simulink model "INS"  (R2018b)
settings: configuration reference "ins_config" (kept outside this file)
undefined symbols (not defined in the file): DiscIntNeverNeededParam, INS_CONST, INS_EXPORT, INS_PARAM
libraries: simulink x99, AP_Math x15, Filter x6, Quaternion x2, Rotation x2
(part 3 of 4)

== system INS/Data_Fusion/AHRS/Correct/Bias_Correction/Onground_Correction ==
  gyr_B_radPs : Inport
  standstill : Inport  Port=2
  Gain : Gain  Gain=2  OutDataTypeStr=single
  Logical Operator : Logic  Operator=NOT  AllPortsSameDT=off  OutDataTypeStr=boolean
  Product : Product  Inputs=3
  Rate Limiter : RateLimiter  RisingSlewLimit=1/600  FallingSlewLimit=-1/3  SampleTimeMode=inherited  InitialCondition=2
  Saturation : Saturate  UpperLimit=1  LowerLimit=1/20
  Saturation1 : Saturate  UpperLimit=3/180*pi  LowerLimit=-3/180*pi
  gyr_bias : Outport
  wires:
  Saturation1/1 -> Product/1
  Gain/1 -> Rate Limiter/1
  Saturation/1 -> Product/3
  Logical Operator/1 -> Gain/1
  gyr_B_radPs/1 -> Saturation1/1
  Product/1 -> gyr_bias/1
  Rate Limiter/1 -> Saturation/1
  standstill/1 -> Product/2, Logical Operator/1

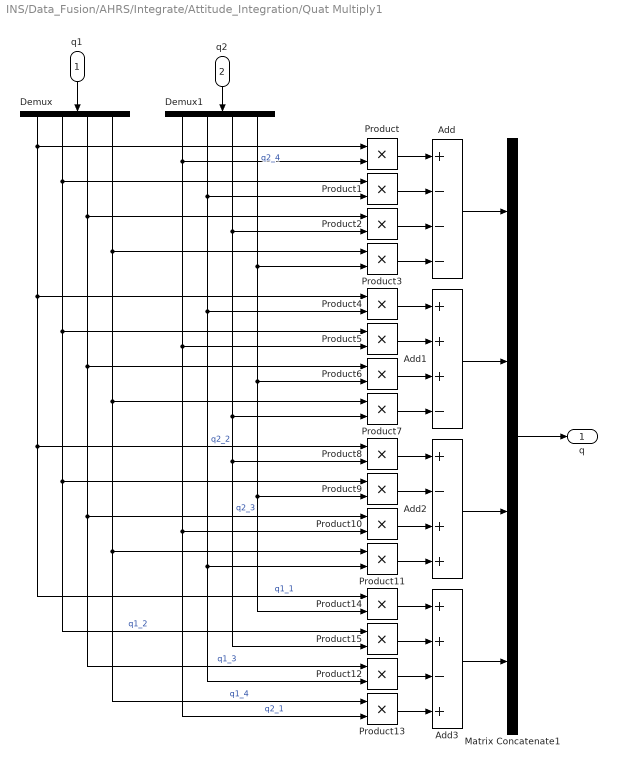
== system INS/Data_Fusion/AHRS/Integrate/Attitude_Integration/Quat Multiply1 ==
  q1 : Inport
  q2 : Inport  Port=2
  Add : Sum  Inputs=+---
  Add1 : Sum  Inputs=+++-
  Add2 : Sum  Inputs=+-++
  Add3 : Sum  Inputs=++-+
  Demux : Demux
  Demux1 : Demux
  Matrix Concatenate1 : Concatenate  NumInputs=4  Mode=Multidimensional array
  Product{,1..15} (16 alike) : Product  RndMeth=Zero
  q : Outport
  wires:
  q1/1 -> Demux/1
  q2/1 -> Demux1/1
  Matrix Concatenate1/1 -> q/1
  Add/1 -> Matrix Concatenate1/1
  Product/1 -> Add/1
  Product1/1 -> Add/2
  Product2/1 -> Add/3
  Product3/1 -> Add/4
  Add1/1 -> Matrix Concatenate1/2
  Product4/1 -> Add1/1
  Product5/1 -> Add1/2
  Product6/1 -> Add1/3
  Product7/1 -> Add1/4
  Product8/1 -> Add2/1
  Product9/1 -> Add2/2
  Product10/1 -> Add2/3
  Product11/1 -> Add2/4
  Product14/1 -> Add3/1
  Product15/1 -> Add3/2
  Product12/1 -> Add3/3
  Product13/1 -> Add3/4
  Add3/1 -> Matrix Concatenate1/4
  Add2/1 -> Matrix Concatenate1/3
  Demux/1 -> Product/1, Product14/1, Product8/1, Product4/1  "q1_1"
  Demux/2 -> Product15/1, Product9/1, Product5/1, Product1/1  "q1_2"
  Demux/3 -> Product12/1, Product10/1, Product6/1, Product2/1  "q1_3"
  Demux/4 -> Product13/1, Product11/1, Product7/1, Product3/1  "q1_4"
  Demux1/4 -> Product14/2, Product9/2, Product6/2, Product3/2  "q2_4"
  Demux1/3 -> Product15/2, Product8/2, Product7/2, Product2/2  "q2_3"
  Demux1/2 -> Product12/2, Product11/2, Product4/2, Product1/2  "q2_2"
  Demux1/1 -> Product13/2, Product10/2, Product5/2, Product/2  "q2_1"

== system INS/Data_Fusion/AHRS/Integrate/Euler_Angle/Euler_Transformations ==
  Oz_B : Inport
  quat_OB : Inport  Port=2
  Demux2 : Demux  Outputs=3
  Gain5 : Gain  Gain=-1
  Saturation1 : Saturate  UpperLimit=0.999  LowerLimit=-0.999
  Trigonometric Function : Trigonometry  Operator=asin
  Trigonometric Function1 : Trigonometry  Operator=atan2
  quat_to_psi : Subsystem
  phi_rad : Outport
  theta_rad : Outport  Port=2
  psi_rad : Outport  Port=3
  wires:
  quat_OB/1 -> quat_to_psi/1(quat)
  Saturation1/1 -> Trigonometric Function/1
  Demux2/1 -> Gain5/1
  Demux2/3 -> Trigonometric Function1/2
  Gain5/1 -> Saturation1/1
  Oz_B/1 -> Demux2/1
  Demux2/2 -> Trigonometric Function1/1
  Trigonometric Function/1 -> theta_rad/1  "theta_rad"
  Trigonometric Function1/1 -> phi_rad/1  "phi_rad"
  quat_to_psi/1(psi) -> psi_rad/1

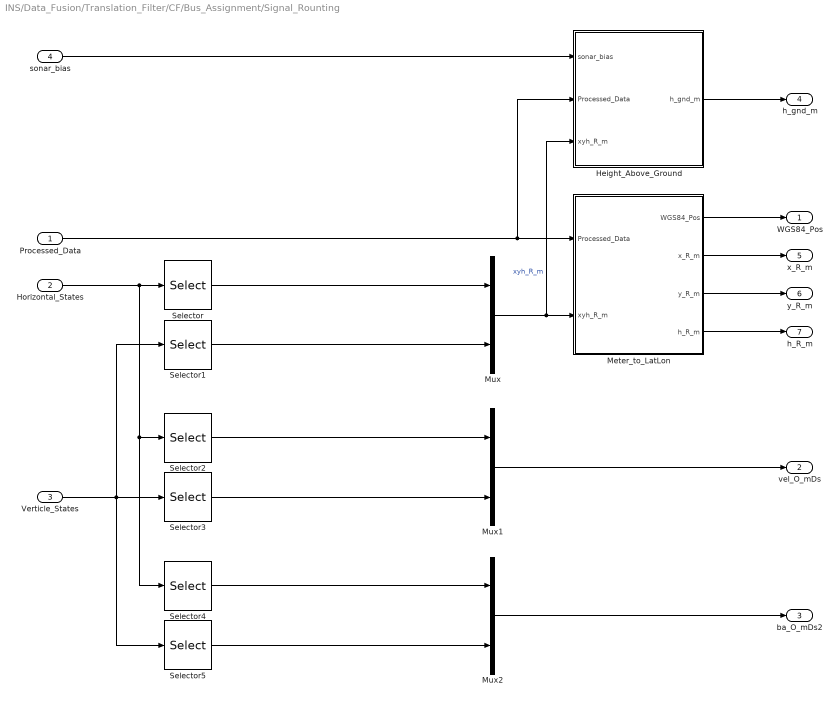
== system INS/Data_Fusion/Translation_Filter/CF/Bus_Assignment/Signal_Rounting ==
  Processed_Data : Inport
  Horizontal_States : Inport  Port=2
  Verticle_States : Inport  Port=3
  sonar_bias : Inport  Port=4
  Height_Above_Ground : Subsystem
  Meter_to_LatLon : Subsystem
  Mux : Mux  Inputs=2
  Mux1 : Mux  Inputs=2
  Mux2 : Mux  Inputs=2
  Selector : Selector  InputPortWidth=6  IndexOptions=Index vector (dialog)  Indices=[1 2]  OutputSizes=1
  Selector1 : Selector  InputPortWidth=3  IndexOptions=Index vector (dialog)  Indices=[1]  OutputSizes=1
  Selector2 : Selector  InputPortWidth=6  IndexOptions=Index vector (dialog)  Indices=[3 4]  OutputSizes=1
  Selector3 : Selector  InputPortWidth=3  IndexOptions=Index vector (dialog)  Indices=[2]  OutputSizes=1
  Selector4 : Selector  InputPortWidth=6  IndexOptions=Index vector (dialog)  Indices=[5 6]  OutputSizes=1
  Selector5 : Selector  InputPortWidth=3  IndexOptions=Index vector (dialog)  Indices=[3]  OutputSizes=1
  WGS84_Pos : Outport
  vel_O_mDs : Outport  Port=2
  ba_O_mDs2 : Outport  Port=3
  h_gnd_m : Outport  Port=4
  x_R_m : Outport  Port=5
  y_R_m : Outport  Port=6
  h_R_m : Outport  Port=7
  wires:
  Mux/1 -> Height_Above_Ground/3(xyh_R_m), Meter_to_LatLon/2(xyh_R_m)  "xyh_R_m"
  Meter_to_LatLon/1(WGS84_Pos) -> WGS84_Pos/1
  Processed_Data/1 -> Height_Above_Ground/2(Processed_Data), Meter_to_LatLon/1(Processed_Data)
  Selector/1 -> Mux/1
  Mux2/1 -> ba_O_mDs2/1
  Selector1/1 -> Mux/2
  Selector4/1 -> Mux2/1
  Selector2/1 -> Mux1/1
  Selector3/1 -> Mux1/2
  Mux1/1 -> vel_O_mDs/1
  Horizontal_States/1 -> Selector/1, Selector2/1, Selector4/1
  Selector5/1 -> Mux2/2
  Verticle_States/1 -> Selector3/1, Selector5/1, Selector1/1
  Height_Above_Ground/1(h_gnd_m) -> h_gnd_m/1
  sonar_bias/1 -> Height_Above_Ground/1(sonar_bias)
  Meter_to_LatLon/4(h_R_m) -> h_R_m/1
  Meter_to_LatLon/2(x_R_m) -> x_R_m/1
  Meter_to_LatLon/3(y_R_m) -> y_R_m/1

== system INS/Data_Fusion/Translation_Filter/CF/Horizontal_Filter/Correct ==
  X_Predict : Inport
  Processed_Data : Inport  Port=2
  Bus Selector : BusSelector  OutputSignals=Sensor_Enable.gps_enable
  GPS_Correct : Subsystem
  Switch : Switch  Criteria=u2 > Threshold
  X_Next : Outport
  wires:
  X_Predict/1 -> GPS_Correct/2(X_Predict), Switch/3
  Processed_Data/1 -> GPS_Correct/1(Processed_Data), Bus Selector/1
  Bus Selector/1 -> GPS_Correct/Enable, Switch/2  "<gps_enable>"
  Switch/1 -> X_Next/1
  GPS_Correct/1(X_Next) -> Switch/1

== system INS/Data_Fusion/Translation_Filter/CF/Horizontal_Filter/Predict ==
  X_Prio : Inport
  Rotation_Data : Inport  Port=2
  Processed_Data : Inport  Port=3
  Propagate : Subsystem
  Update : Subsystem
  X_Predict : Outport
  wires:
  X_Prio/1 -> Propagate/1(X_prio)
  Processed_Data/1 -> Propagate/2(Processed_Data)
  Propagate/1(X) -> Update/1(X_Prio)
  Rotation_Data/1 -> Update/2(Rotation_Data)
  Update/1(X_Predict) -> X_Predict/1

== system INS/Data_Fusion/Translation_Filter/CF/Verticle_Filter/Correct ==
  X_Predict : Inport
  Processed_Data : Inport  Port=2
  Baro_Correct : Subsystem
  GPS_Correct : Subsystem
  X_Next : Outport
  wires:
  Processed_Data/1 -> GPS_Correct/2(Processed_Data), Baro_Correct/2(Processed_Data)
  X_Predict/1 -> Baro_Correct/1(X_Predict)
  Baro_Correct/1(X_Next) -> GPS_Correct/1(X_Predict)
  GPS_Correct/1(X_Next) -> X_Next/1

== system INS/Data_Fusion/Translation_Filter/CF/Verticle_Filter/Predict ==
  X_Prio : Inport
  Rotation_Data : Inport  Port=2
  Processed_Data : Inport  Port=3
  Propagate : Subsystem
  Update : Subsystem
  X_Predict : Outport
  wires:
  X_Prio/1 -> Propagate/1(X_Prio)
  Processed_Data/1 -> Propagate/2(Processed_Data)
  Propagate/1(X) -> Update/1(X_Prio)
  Rotation_Data/1 -> Update/2(Rotation_Data)
  Update/1(X_Predict) -> X_Predict/1

== system INS/Data_Fusion/Translation_Filter/Process/Process_Data/Init_Condition ==
  Validity : Inport
  global_reset : Inport  Port=2
  Sensor_Meas : Inport  Port=3
  Rotation_Data : Inport  Port=4
  Translation_Data : Inport  Port=5
  Bus Creator : BusCreator  Inputs=4
  Bus_Selection : Subsystem
  Pos_Reset : Subsystem
  WGS84_Reference : Subsystem
  Init_Condition : Outport
  wires:
  WGS84_Reference/1(WGS84_Ref) -> Bus Creator/3  "WGS84_Ref"
  Rotation_Data/1 -> Pos_Reset/1(Rotation_Data)
  Bus_Selection/2(WGS84_position) -> WGS84_Reference/4(WGS84_position)
  Bus_Selection/1(WGS84_derivatives) -> WGS84_Reference/3(WGS84_derivatives)
  Pos_Reset/1(pos_reset) -> Bus Creator/1  "pos_reset"
  Sensor_Meas/1 -> Bus_Selection/1(Sensor_Meas)
  Validity/1 -> Pos_Reset/3(Validity), Bus Creator/4, WGS84_Reference/1(Validity)  "Pos_Validity"
  global_reset/1 -> Pos_Reset/2(global_reset)
  Pos_Reset/2(height_reset) -> Bus Creator/2  "height_reset"
  Bus Creator/1 -> Init_Condition/1
  Translation_Data/1 -> WGS84_Reference/2(Translation_Data)

== system INS/Data_Fusion/Translation_Filter/Process/Process_Data/Sensor_Enable ==
  Sensor_Status : Inport
  Bus Creator : BusCreator  Inputs=5
  Bus Selector : BusSelector  OutputSignals=GPS_Status.pos_quality,GPS_Status.spd_quality,GPS_Status.GPS_vaid,OptFlow_Status.opt_flow_valid,Sonar_Status.sonar_valid,Baro_Status.baro_valid
  Sensor_Horizontal_Select : Subsystem
  Sensor_Vertical_Select : Subsystem
  Sensor_Enable : Outport
  wires:
  Bus Selector/3 -> Sensor_Vertical_Select/3(gps_valid), Sensor_Horizontal_Select/3(gps_valid)  "<GPS_vaid>"
  Bus Selector/1 -> Sensor_Vertical_Select/1(gps_pos_quality), Sensor_Horizontal_Select/1(gps_pos_quality)  "<pos_quality>"
  Sensor_Status/1 -> Bus Selector/1
  Sensor_Horizontal_Select/1(gps_enable) -> Bus Creator/1  "gps_enable"
  Sensor_Vertical_Select/2(sonar_enable) -> Bus Creator/4  "sonar_enable"
  Sensor_Vertical_Select/1(gps_hgt_enable) -> Bus Creator/3  "gps_height_enable"
  Bus Creator/1 -> Sensor_Enable/1
  Sensor_Vertical_Select/3(baro_enable) -> Bus Creator/5  "baro_enable"
  Bus Selector/4 -> Sensor_Horizontal_Select/4(opt_flow_valid)  "<opt_flow_valid>"
  Sensor_Horizontal_Select/2(op_flow_enable) -> Bus Creator/2  "opt_flow_enable"
  Bus Selector/2 -> Sensor_Vertical_Select/2(gps_spd_quality), Sensor_Horizontal_Select/2(gps_spd_quality)  "<spd_quality>"
  Bus Selector/6 -> Sensor_Vertical_Select/5(baro_valid)  "<baro_valid>"
  Bus Selector/5 -> Sensor_Vertical_Select/4(sonar_valid)  "<sonar_valid>"

== system INS/Data_Fusion/Translation_Filter/Process/Process_Data/Sensor_Valid ==
  Sensor_Status : Inport
  Bus Creator : BusCreator  Inputs=4
  Position_Validity : Subsystem
  Validity : Outport
  wires:
  Sensor_Status/1 -> Position_Validity/1(Sensor_Status)
  Position_Validity/1(lon_lat_valid) -> Bus Creator/1  "lon_lat_valid"
  Position_Validity/2(xy_R_valid) -> Bus Creator/2  "xy_R_valid"
  Position_Validity/3(altitude_valid) -> Bus Creator/3  "altitude_valid"
  Position_Validity/4(h_R_valid) -> Bus Creator/4  "h_R_valid"
  Bus Creator/1 -> Validity/1

== system INS/Data_Fusion/Translation_Filter/Process/Sensor_Meas/Baro_Process ==
  Sensor_Data : Inport
  Bus Creator : BusCreator  Inputs=2
  Bus Selector1 : BusSelector  OutputSignals=Baro_Data.timestamp,Baro_Data.h_R_m
  Signal Copy : SignalConversion  OverrideOpt=off
  Signal Copy1 : SignalConversion  OverrideOpt=off
  Baro_Meas : Outport
  wires:
  Sensor_Data/1 -> Bus Selector1/1
  Bus Selector1/2 -> Signal Copy1/1  "<h_R_m>"
  Bus Creator/1 -> Baro_Meas/1
  Bus Selector1/1 -> Signal Copy/1  "<timestamp>"
  Signal Copy/1 -> Bus Creator/1  "timestamp_ms"
  Signal Copy1/1 -> Bus Creator/2  "h_R_m"

== system INS/Data_Fusion/Translation_Filter/Process/Sensor_Meas/GPS_Process ==
  Sensor_Data : Inport
  Bus Creator : BusCreator  Inputs=12
  Bus Selector : BusSelector  OutputSignals=GPS_Data.signal6,GPS_Data.signal7,GPS_Data.dz_dh,GPS_Data.mue_rad,GPS_Data.lambda_rad,GPS_Data.height_m,GPS_Data.vn_mPs,GPS_Data.ve_mPs,GPS_Data.vd_mPs,GPS_Data.timestamp_ms,GPS_Data.GPS_reset,GPS_Data.sqd_quality,GPS_Data.pos_quality
  Logical Operator : Logic  Operator=NOT  AllPortsSameDT=off  OutDataTypeStr=boolean
  Multiply : Product
  Multiply1 : Product
  Signal Conversion{,1..9} (10 alike) : SignalConversion  OverrideOpt=off
  GPS_Meas : Outport
  wires:
  Multiply1/1 -> Bus Creator/12  "pos_quality"
  Logical Operator/1 -> Multiply1/1, Multiply/1
  Multiply/1 -> Bus Creator/11  "spd_quality"
  Bus Selector/13 -> Multiply1/2  "<pos_quality>"
  Bus Selector/12 -> Multiply/2  "<sqd_quality>"
  Bus Selector/11 -> Logical Operator/1  "<GPS_reset>"
  Signal Conversion9/1 -> Bus Creator/10  "timestamp_ms"
  Signal Conversion8/1 -> Bus Creator/9  "vel_D_mPs"
  Signal Conversion7/1 -> Bus Creator/8  "vel_E_mPs"
  Signal Conversion6/1 -> Bus Creator/7  "vel_N_mPs"
  Signal Conversion5/1 -> Bus Creator/6  "h_m"
  Signal Conversion4/1 -> Bus Creator/5  "lambda_rad"
  Signal Conversion3/1 -> Bus Creator/4  "mue_rad"
  Signal Conversion2/1 -> Bus Creator/3  "dz_dh"
  Signal Conversion1/1 -> Bus Creator/2  "dy_dlambda"
  Signal Conversion/1 -> Bus Creator/1  "dx_dmue"
  Bus Selector/10 -> Signal Conversion9/1  "<timestamp_ms>"
  Bus Selector/9 -> Signal Conversion8/1  "<vd_mPs>"
  Bus Selector/8 -> Signal Conversion7/1  "<ve_mPs>"
  Bus Selector/7 -> Signal Conversion6/1  "<vn_mPs>"
  Bus Selector/6 -> Signal Conversion5/1  "<height_m>"
  Bus Selector/5 -> Signal Conversion4/1  "<lambda_rad>"
  Bus Selector/4 -> Signal Conversion3/1  "<mue_rad>"
  Bus Selector/3 -> Signal Conversion2/1  "<dz_dh>"
  Bus Selector/2 -> Signal Conversion1/1  "<signal7>"
  Bus Selector/1 -> Signal Conversion/1  "<signal6>"
  Bus Creator/1 -> GPS_Meas/1
  Sensor_Data/1 -> Bus Selector/1

== system INS/Data_Fusion/Translation_Filter/Process/Sensor_Meas/OpticalFlow_Process ==
  Sensor_Data : Inport
  Bus Creator : BusCreator  Inputs=3
  Bus Selector1 : BusSelector  OutputSignals=VisionFlow_Data.timestamp_ms,VisionFlow_Data.vel_x_O_mDs,VisionFlow_Data.vel_y_O_mDs
  Signal Copy : SignalConversion  OverrideOpt=off
  Signal Copy1 : SignalConversion  OverrideOpt=off
  Signal Copy2 : SignalConversion  OverrideOpt=off
  OptFlow_Meas : Outport
  wires:
  Sensor_Data/1 -> Bus Selector1/1
  Bus Creator/1 -> OptFlow_Meas/1
  Signal Copy/1 -> Bus Creator/1  "timestamp_ms"
  Signal Copy1/1 -> Bus Creator/2  "vel_x_O"
  Bus Selector1/1 -> Signal Copy/1  "<timestamp_ms>"
  Bus Selector1/2 -> Signal Copy1/1  "<vel_x_O_mDs>"
  Bus Selector1/3 -> Signal Copy2/1  "<vel_y_O_mDs>"
  Signal Copy2/1 -> Bus Creator/3  "vel_y_O"

== system INS/Data_Fusion/Translation_Filter/Process/Sensor_Meas/Sonar_Process ==
  Sensor_Data : Inport
  Rotation_Data : Inport  Port=2
  Bus Creator : BusCreator  Inputs=2
  Bus Selector : BusSelector  OutputSignals=phi_rad,theta_rad
  Bus Selector1 : BusSelector  OutputSignals=Sonar_Data.timestamp_ms,Sonar_Data.distance_m
  Cos : Trigonometry  Operator=cos
  Cos1 : Trigonometry  Operator=cos
  Multiply : Product  Inputs=3
  Signal Copy : SignalConversion  OverrideOpt=off
  Sonar_Meas : Outport
  wires:
  Rotation_Data/1 -> Bus Selector/1
  Sensor_Data/1 -> Bus Selector1/1
  Bus Selector1/2 -> Multiply/1  "<distance_m>"
  Bus Selector/1 -> Cos/1  "<phi_rad>"
  Bus Selector/2 -> Cos1/1  "<theta_rad>"
  Cos/1 -> Multiply/2
  Cos1/1 -> Multiply/3
  Multiply/1 -> Bus Creator/2  "distance_m"
  Bus Creator/1 -> Sonar_Meas/1
  Bus Selector1/1 -> Signal Copy/1  "<timestamp_ms>"
  Signal Copy/1 -> Bus Creator/1  "timestamp_ms"

== system INS/Data_Fusion/Translation_Filter/Process/Sensor_Status/Baro_Status ==
  Sensor_Data : Inport
  Bus Creator : BusCreator  Inputs=1
  Bus Selector : BusSelector  OutputSignals=Baro_Data.baro_valid
  Signal Conversion1 : SignalConversion  OverrideOpt=off
  Baro_Status : Outport
  wires:
  Bus Selector/1 -> Signal Conversion1/1  "<baro_valid>"
  Bus Creator/1 -> Baro_Status/1
  Sensor_Data/1 -> Bus Selector/1
  Signal Conversion1/1 -> Bus Creator/1  "baro_valid"

== system INS/Data_Fusion/Translation_Filter/Process/Sensor_Status/GPS_Status ==
  Sensor_Data : Inport
  Bus Creator : BusCreator  Inputs=3
  Bus Selector : BusSelector  OutputSignals=GPS_Data.GPS_reset,GPS_Data.sqd_quality,GPS_Data.pos_quality
  Logical Operator : Logic  Operator=NOT  AllPortsSameDT=off  OutDataTypeStr=boolean
  Signal Conversion : SignalConversion  OverrideOpt=off
  Signal Conversion1 : SignalConversion  OverrideOpt=off
  GPS_Status : Outport
  wires:
  Bus Creator/1 -> GPS_Status/1
  Signal Conversion1/1 -> Bus Creator/3  "pos_quality"
  Signal Conversion/1 -> Bus Creator/2  "spd_quality"
  Logical Operator/1 -> Bus Creator/1  "GPS_vaid"
  Bus Selector/3 -> Signal Conversion1/1  "<pos_quality>"
  Bus Selector/2 -> Signal Conversion/1  "<sqd_quality>"
  Bus Selector/1 -> Logical Operator/1  "<GPS_reset>"
  Sensor_Data/1 -> Bus Selector/1

== system INS/Data_Fusion/Translation_Filter/Process/Sensor_Status/OpticalFlow_Status ==
  Sensor_Data : Inport
  Bus Creator : BusCreator  Inputs=1
  Bus Selector : BusSelector  OutputSignals=VisionFlow_Data.valid
  Signal Conversion1 : SignalConversion  OverrideOpt=off
  OptFlow_Status : Outport
  wires:
  Bus Selector/1 -> Signal Conversion1/1  "<valid>"
  Bus Creator/1 -> OptFlow_Status/1
  Sensor_Data/1 -> Bus Selector/1
  Signal Conversion1/1 -> Bus Creator/1  "opt_flow_valid"

== system INS/Data_Fusion/Translation_Filter/Process/Sensor_Status/Sonar_Status ==
  Sensor_Data : Inport
  Bus Creator : BusCreator  Inputs=1
  Bus Selector : BusSelector  OutputSignals=Sonar_Data.sonar_valid
  Signal Conversion1 : SignalConversion  OverrideOpt=off
  Sonar_Status : Outport
  wires:
  Signal Conversion1/1 -> Bus Creator/1  "sonar_valid"
  Sensor_Data/1 -> Bus Selector/1
  Bus Creator/1 -> Sonar_Status/1
  Bus Selector/1 -> Signal Conversion1/1  "<sonar_valid>"

== system INS/Sensor_Process/GPS_Process/GPS_Status_and_Quality/GPS_Status/Init_Condition ==
  valid : Inport
  Compare To Constant3 : simulink/Logic and Bit Operations/Compare To Constant  relop=>=  const=1000  OutDataTypeStr=boolean
  Saturation : Saturate  UpperLimit=2000  LowerLimit=0
  Sum : Sum  Inputs=|++  OutDataTypeStr=int32
  Unit Delay : UnitDelay  SampleTime=-1
  initialized : Outport
  wires:
  Compare To Constant3/1 -> initialized/1  "initialized"
  Sum/1 -> Saturation/1
  Unit Delay/1 -> Compare To Constant3/1, Sum/2
  Saturation/1 -> Unit Delay/1
  valid/1 -> Sum/1

== system INS/Sensor_Process/Mag_Process/Magnetometer/Quality_Indication/Mag_Quality_Estimate ==
  nominal_Inclination_deg : Inport
  mag_normalized_O : Inport  Port=2
  Inclination_Quality_Estimate : Subsystem
  Intensity_Quality_Estimate : Subsystem
  MinMax : MinMax  Inputs=2
  mag_quality : Outport
  wires:
  Intensity_Quality_Estimate/1(intensity_quality) -> MinMax/2  "intensity_quality"
  nominal_Inclination_deg/1 -> Inclination_Quality_Estimate/1(nominal_inc_deg)
  Inclination_Quality_Estimate/1(inclination_quality) -> MinMax/1  "inclination_quality"
  mag_normalized_O/1 -> Inclination_Quality_Estimate/2(mag_normalized_O), Intensity_Quality_Estimate/1(mag_normalized_O)
  MinMax/1 -> mag_quality/1

== system INS/Sensor_Process/Mag_Process/Magnetometer/WMM_Compensation/psi_to_Mz ==
  psi : Inport
  Constant : Constant  OutDataTypeStr=Inherit: Inherit via back propagation
  Constant{1..4} (4 alike) : Constant  Value=0  OutDataTypeStr=Inherit: Inherit via back propagation
  Gain : Gain  Gain=-1
  Trigonometric Function : Trigonometry
  Trigonometric Function1 : Trigonometry  Operator=cos
  Trigonometric Function2 : Trigonometry
  Trigonometric Function3 : Trigonometry  Operator=cos
  Vector Concatenate : Concatenate  NumInputs=3  Mode=Multidimensional array  ConcatenateDimension=2
  Vector Concatenate1 : Concatenate  NumInputs=3  Mode=Multidimensional array
  Vector Concatenate2 : Concatenate  NumInputs=3  Mode=Multidimensional array
  Vector Concatenate3 : Concatenate  NumInputs=3  Mode=Multidimensional array
  Mz : Outport
  wires:
  Vector Concatenate/1 -> Mz/1
  Vector Concatenate1/1 -> Vector Concatenate/1
  Trigonometric Function3/1 -> Vector Concatenate2/2
  Constant4/1 -> Vector Concatenate2/3
  Trigonometric Function1/1 -> Vector Concatenate1/1
  Vector Concatenate2/1 -> Vector Concatenate/2
  Vector Concatenate3/1 -> Vector Concatenate/3
  Trigonometric Function2/1 -> Gain/1
  psi/1 -> Trigonometric Function3/1, Trigonometric Function2/1, Trigonometric Function/1, Trigonometric Function1/1
  Constant/1 -> Vector Concatenate3/3
  Constant3/1 -> Vector Concatenate1/3
  Trigonometric Function/1 -> Vector Concatenate1/2
  Gain/1 -> Vector Concatenate2/1
  Constant2/1 -> Vector Concatenate3/1
  Constant1/1 -> Vector Concatenate3/2

== system INS/Data_Fusion/AHRS/Correct/Att_Correction/Attitude_Correct/Acc_Correct ==
  acc_meas_O_mPs2 : Inport
  acc_ob_valid : Inport  Port=2
  acc_est_O_mPs2 : Inport  Port=3
  Heading_Correct : Subsystem
  Sum : Sum  Inputs=|++
  Verticle_Correct : Subsystem
  att_error_O : Outport
  wires:
  acc_ob_valid/1 -> Heading_Correct/3(acc_ob_valid)
  Verticle_Correct/1(vert_correct) -> Sum/1
  Heading_Correct/1(hor_correct) -> Sum/2
  Sum/1 -> att_error_O/1
  acc_meas_O_mPs2/1 -> Heading_Correct/2(sfor_O_meas_mPs2), Verticle_Correct/2(acc_meas_O_mPs2)
  acc_est_O_mPs2/1 -> Verticle_Correct/1(acc_est_O_mPs2), Heading_Correct/1(sfor_O_est_mPs2)

== system INS/Data_Fusion/AHRS/Correct/Att_Correction/Attitude_Correct/Estimated_Acc ==
  delay : Inport
  Sensor_Data : Inport  Port=2
  Rotation_Data : Inport  Port=3
  2_Order_Butter_LPF : Filter/2_Order_Butter_LPF  wn=30*2*pi  ksi=0.707
  Bus Selector : BusSelector  OutputSignals=IMU_Data.acc_B_mPs2
  Bus Selector1 : BusSelector  OutputSignals=M_OB
  Delay : Delay  DelayLengthSource=Input port  DelayLengthUpperLimit=200
      settings: InputPortMap=u0,p1
  Multiply : Product  Multiplication=Matrix(*)
  acc_O_est_mPs2 : Outport
  wires:
  2_Order_Butter_LPF/1 -> Delay/1
  Multiply/1 -> 2_Order_Butter_LPF/1  "acc_O"
  Bus Selector/1 -> Multiply/2  "<acc_B_mPs2>"
  Bus Selector1/1 -> Multiply/1  "<M_OB>"
  Rotation_Data/1 -> Bus Selector1/1
  Sensor_Data/1 -> Bus Selector/1
  delay/1 -> Delay/2
  Delay/1 -> acc_O_est_mPs2/1

== system INS/Data_Fusion/AHRS/Correct/Att_Correction/Attitude_Correct/Measured_Acc ==
  Sensor_Data : Inport
  Detect Increase : simulink/Logic and Bit Operations/Detect Increase  vinit=0.0  OutDataTypeStr=boolean
  GPS_Acc_Observer : Subsystem
  Observer_Sensor : Subsystem
  OpticalFlow_Acc_Observer : Subsystem
  Routing : Subsystem
  meas_acc_O_mPs2 : Outport
  acc_ob_valid : Outport  Port=2
  acc_delay : Outport  Port=3
  wires:
  Routing/2(acc_ob_valid) -> acc_ob_valid/1
  Routing/3(acc_delay) -> acc_delay/1
  Routing/1(meas_acc_O_mPs2) -> meas_acc_O_mPs2/1
  GPS_Acc_Observer/1(GPS_acc_O_mPs2) -> Routing/2(GPS_acc_O_mPs2)
  Observer_Sensor/2(GPS_vel_O_mPs) -> GPS_Acc_Observer/2(GPS_vel_O_mPs)
  Observer_Sensor/1(gps_ob_enable) -> Detect Increase/1, GPS_Acc_Observer/Enable, Routing/1(gps_ob_enable)  "gps_ob_enable"
  Sensor_Data/1 -> Observer_Sensor/1(Sensor_Data)
  Observer_Sensor/4(opt_flow_vel_O_mPs) -> OpticalFlow_Acc_Observer/1(OptFlow_vel_O_mDs)
  Observer_Sensor/3(opt_flow_ob_enable) -> OpticalFlow_Acc_Observer/Enable, Routing/3(opt_flow_ob_enable)
  OpticalFlow_Acc_Observer/1(OptFlow_acc_O_mPs2) -> Routing/4(opt_flow_acc_O_mPs2)
  Detect Increase/1 -> GPS_Acc_Observer/1(reset)

== system INS/Data_Fusion/AHRS/Correct/Att_Correction/Heading_Correction/Enable ==
  Mag_quality : Inport
  Mag_Enable : Inport  Port=2
  Logical Operator : Logic  AllPortsSameDT=off  OutDataTypeStr=boolean
  Relay1 : Relay  OnSwitchValue=0.3  OffSwitchValue=0.2
  Mag_Correct_Enable : Outport
  wires:
  Relay1/1 -> Logical Operator/2
  Mag_quality/1 -> Relay1/1
  Mag_Enable/1 -> Logical Operator/1
  Logical Operator/1 -> Mag_Correct_Enable/1

== system INS/Data_Fusion/AHRS/Correct/Att_Correction/Heading_Correction/Mag_Correction ==
  M_OB : Inport
  mag_B : Inport  Port=2
  Mag_Correct_Enable : Inport  Port=3
  MX Product3 : Product  Inputs=3  RndMeth=Simplest
  MX Product4 : Product  Multiplication=Matrix(*)  RndMeth=Simplest
  Selector2 : Selector  NumberOfDimensions=2  InputPortWidth=3  IndexOptions=Index vector (dialog),Index vector (dialog)  Indices=[3],[1 2 3]  OutputSizes=1,1
  Selector4 : Selector  NumberOfDimensions=2  InputPortWidth=3  IndexOptions=Index vector (dialog),Index vector (dialog)  Indices=[2],[1 2 3]  OutputSizes=1,1
  Transpose2 : Math  Operator=transpose  SaturateOnIntegerOverflow=on
  mag_correct_gain : Gain  Gain=-0.2  OutDataTypeStr=Inherit: Same as input
  mag_corr_O : Outport
  wires:
  MX Product3/1 -> mag_corr_O/1
  Selector4/1 -> MX Product4/1
  mag_B/1 -> MX Product4/2
  Transpose2/1 -> MX Product3/1  "Bz_O"
  Mag_Correct_Enable/1 -> MX Product3/3
  MX Product4/1 -> mag_correct_gain/1  "my_O"
  M_OB/1 -> Selector2/1, Selector4/1
  mag_correct_gain/1 -> MX Product3/2
  Selector2/1 -> Transpose2/1

== system INS/Data_Fusion/AHRS/Correct/Att_Correction/Heading_Correction/Subsystem ==
  M_OB : Inport
  mag_B : Inport  Port=2
  Rotation_Data : Inport  Port=3
  Add : Sum
  Atan2 : Trigonometry  Operator=atan2
  Bus Selector : BusSelector  OutputSignals=psi_rad
  Demux : Demux  Outputs=3
  Gain : Gain  Gain=-1
  MX Product1 : Product  Multiplication=Matrix(*)  RndMeth=Simplest
  Terminator : Terminator
  Terminator1 : Terminator
  wires:
  Demux/3 -> Terminator1/1
  Atan2/1 -> Add/1
  Demux/1 -> Atan2/2
  MX Product1/1 -> Demux/1  "my_O"
  Gain/1 -> Atan2/1
  Add/1 -> Terminator/1  "mag_heading"
  Rotation_Data/1 -> Bus Selector/1
  Bus Selector/1 -> Add/2  "<psi_rad>"
  Demux/2 -> Gain/1
  mag_B/1 -> MX Product1/2
  M_OB/1 -> MX Product1/1

== system INS/Data_Fusion/AHRS/Integrate/Euler_Angle/Euler_Transformations/quat_to_psi ==
  quat : Inport
  Add : Sum  Inputs=++--
  Add1 : Sum
  Demux1 : Demux
  Demux2 : Demux
  Gain : Gain  Gain=2  OutDataTypeStr=Inherit: Same as input
  Product : Product  RndMeth=Zero
  Product1 : Product  RndMeth=Zero
  Product2 : Product  RndMeth=Zero
  Trigonometric Function1 : Trigonometry  Operator=atan2  OutputSignalType=real
  psi : Outport
  wires:
  Demux1/2 -> Product1/1  "q2"
  Product2/1 -> Add1/2
  Product1/1 -> Add1/1
  Gain/1 -> Trigonometric Function1/1
  Add1/1 -> Gain/1
  Add/1 -> Trigonometric Function1/2
  Demux1/1 -> Product2/1  "q1"
  Demux1/3 -> Product1/2  "q3"
  Demux1/4 -> Product2/2  "q4"
  Demux2/4 -> Add/4  "q4^2"
  Demux2/3 -> Add/3  "q3^2"
  Demux2/2 -> Add/2  "q2^2"
  Demux2/1 -> Add/1  "q1^2"
  Product/1 -> Demux2/1
  Trigonometric Function1/1 -> psi/1
  quat/1 -> Product/2, Product/1, Demux1/1

== system INS/Data_Fusion/Translation_Filter/CF/Bus_Assignment/Signal_Rounting/Height_Above_Ground ==
  sonar_bias : Inport
  Processed_Data : Inport  Port=2
  xyh_R_m : Inport  Port=3
  Bus Selector : BusSelector  OutputSignals=Sensor_Status.Sonar_Status.sonar_valid
  Constant : Constant  Value=-1  OutDataTypeStr=single
  Selector6 : Selector  InputPortWidth=3  IndexOptions=Index vector (dialog)  Indices=3  OutputSizes=1
  Sum : Sum  Inputs=|+-
  Switch : Switch  Criteria=u2 > Threshold
  h_gnd_m : Outport
  wires:
  xyh_R_m/1 -> Selector6/1
  Selector6/1 -> Sum/1
  sonar_bias/1 -> Sum/2
  Sum/1 -> Switch/1
  Processed_Data/1 -> Bus Selector/1
  Bus Selector/1 -> Switch/2  "<sonar_valid>"
  Constant/1 -> Switch/3
  Switch/1 -> h_gnd_m/1

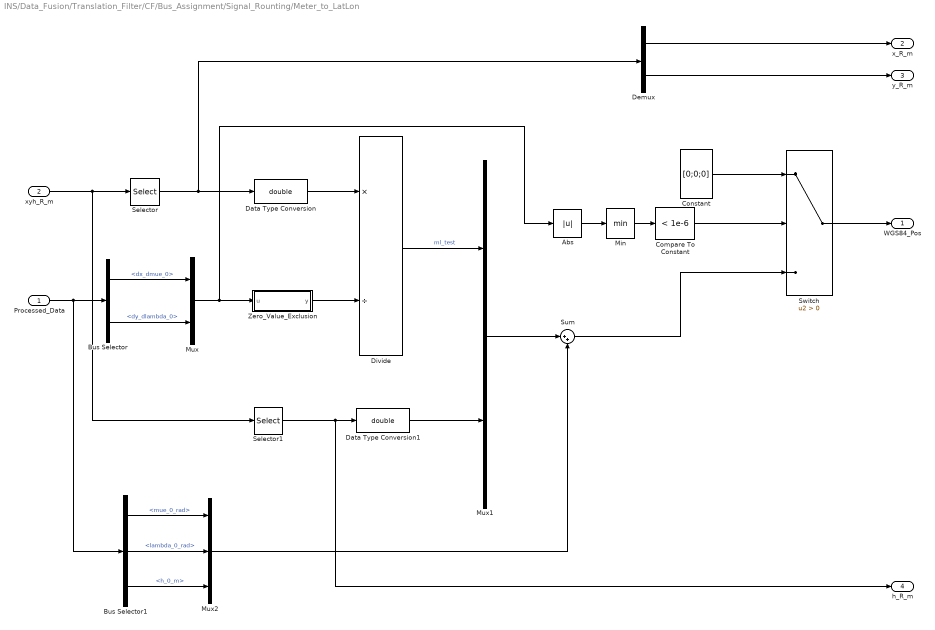
== system INS/Data_Fusion/Translation_Filter/CF/Bus_Assignment/Signal_Rounting/Meter_to_LatLon ==
  Processed_Data : Inport
  xyh_R_m : Inport  Port=2
  Abs : Abs
  Bus Selector : BusSelector  OutputSignals=Init_Condition.WGS84_Ref.WGS84_derivatives_ref.dx_dmue_0,Init_Condition.WGS84_Ref.WGS84_derivatives_ref.dy_dlambda_0
  Bus Selector1 : BusSelector  OutputSignals=Init_Condition.WGS84_Ref.WGS84_pos_ref.mue_0_rad,Init_Condition.WGS84_Ref.WGS84_pos_ref.lambda_0_rad,Init_Condition.WGS84_Ref.WGS84_pos_ref.h_0_m
  Compare To Constant : simulink/Logic and Bit Operations/Compare To Constant  relop=<  const=1e-6  OutDataTypeStr=boolean
  Constant : Constant  Value=[0;0;0]  VectorParams1D=off
  Data Type Conversion : DataTypeConversion  OutDataTypeStr=double
  Data Type Conversion1 : DataTypeConversion  OutDataTypeStr=double
  Demux : Demux  Outputs=2
  Divide : Product  Inputs=*/
  Min : MinMax
  Mux : Mux  Inputs=2
  Mux1 : Mux  Inputs=2
  Mux2 : Mux  Inputs=3
  Selector : Selector  InputPortWidth=3  IndexOptions=Index vector (dialog)  Indices=[1 2]  OutputSizes=1
  Selector1 : Selector  InputPortWidth=3  IndexOptions=Index vector (dialog)  Indices=[3]  OutputSizes=1
  Sum : Sum  Inputs=|++
  Switch : Switch  Criteria=u2 > Threshold
  Zero_Value_Exclusion : Subsystem  mask{thr=1e-6}
      mask prompts: thr "Threshold"
      mask Display: disp('Exclude Zero');
  WGS84_Pos : Outport
  x_R_m : Outport  Port=2
  y_R_m : Outport  Port=3
  h_R_m : Outport  Port=4
  wires:
  Switch/1 -> WGS84_Pos/1
  Constant/1 -> Switch/1
  Compare To Constant/1 -> Switch/2
  Min/1 -> Compare To Constant/1
  Sum/1 -> Switch/3
  Mux2/1 -> Sum/2
  Mux1/1 -> Sum/1
  Bus Selector1/3 -> Mux2/3  "<h_0_m>"
  Bus Selector1/2 -> Mux2/2  "<lambda_0_rad>"
  Bus Selector1/1 -> Mux2/1  "<mue_0_rad>"
  Data Type Conversion1/1 -> Mux1/2
  Selector1/1 -> h_R_m/1, Data Type Conversion1/1
  Data Type Conversion/1 -> Divide/1
  Divide/1 -> Mux1/1  "ml_test"
  Selector/1 -> Demux/1, Data Type Conversion/1
  Zero_Value_Exclusion/1(y) -> Divide/2
  xyh_R_m/1 -> Selector1/1, Selector/1
  Mux/1 -> Zero_Value_Exclusion/1(u), Abs/1
  Bus Selector/2 -> Mux/2  "<dy_dlambda_0>"
  Bus Selector/1 -> Mux/1  "<dx_dmue_0>"
  Processed_Data/1 -> Bus Selector/1, Bus Selector1/1
  Abs/1 -> Min/1
  Demux/1 -> x_R_m/1
  Demux/2 -> y_R_m/1

== system INS/Data_Fusion/Translation_Filter/CF/Horizontal_Filter/Correct/GPS_Correct ==
  Processed_Data : Inport
  X_Predict : Inport  Port=2
  Enable : EnablePort
  Bus Selector : BusSelector  OutputSignals=Init_Condition.pos_reset
  Bus Selector1 : BusSelector  OutputSignals=Sensor_Meas.GPS_Meas.timestamp_ms
  Detect Change : simulink/Logic and Bit Operations/Detect Change  vinit=0  OutDataTypeStr=boolean
  Holder : Subsystem
  Logical Operator : Logic  Operator=OR  AllPortsSameDT=off  OutDataTypeStr=boolean
  Measurement : Subsystem
  Observation : Subsystem
  Scaling : Subsystem
  Sum : Sum  Inputs=|-+
  Sum1 : Sum  Inputs=++|
  X_Next : Outport
  wires:
  Observation/1(HX) -> Sum/1  "GPS_HX"
  Measurement/1(Z) -> Sum/2  "GPS_Z"
  Processed_Data/1 -> Bus Selector/1, Measurement/2(Processed_Data), Bus Selector1/1
  Sum/1 -> Scaling/1(y)
  Bus Selector1/1 -> Detect Change/1  "<timestamp_ms>"
  Holder/1(out) -> Sum1/2
  Sum1/1 -> X_Next/1
  X_Predict/1 -> Observation/1(X), Measurement/1(X), Sum1/1
  Bus Selector/1 -> Observation/2(reset)  "<pos_reset>"
  Logical Operator/1 -> Holder/2(update)
  Detect Change/1 -> Logical Operator/2
  Measurement/2(bias_update) -> Logical Operator/1
  Scaling/1(X_error) -> Holder/1(in)

== system INS/Data_Fusion/Translation_Filter/CF/Horizontal_Filter/Predict/Propagate ==
  X_prio : Inport
  Processed_Data : Inport  Port=2
  Bus Selector : BusSelector  OutputSignals=Init_Condition.pos_reset
  Delay : Delay  DelayLength=1
  States_Init : Subsystem
  Switch : Switch  Criteria=u2 > Threshold
  X : Outport
  wires:
  Delay/1 -> Switch/3
  States_Init/1(X_0) -> Switch/1
  Switch/1 -> X/1
  Bus Selector/1 -> Switch/2  "<pos_reset>"
  Processed_Data/1 -> Bus Selector/1, States_Init/1(Processed_Data)
  X_prio/1 -> Delay/1

== system INS/Data_Fusion/Translation_Filter/CF/Horizontal_Filter/Predict/Update ==
  X_Prio : Inport
  Rotation_Data : Inport  Port=2
  Add : Sum  Inputs=-+
  Bus Selector2 : BusSelector  OutputSignals=M_OB,acc_B_mDs2
  Constant : Constant  Value=[0;0]  OutDataTypeStr=single
  Gain : Gain  Gain=INS_CONST.dt  OutDataTypeStr=Inherit: Same as input
  Multiply : Product  Multiplication=Matrix(*)
  Mux : Mux  Inputs=3
  Reshape : Reshape  OutputDimensionality=Customize  OutputDimensions=[6,1]
  Selector : Selector  InputPortWidth=3  IndexOptions=Index vector (dialog)  Indices=[1 2]  OutputSizes=1
  Selector1 : Selector  InputPortWidth=6  IndexOptions=Index vector (dialog)  Indices=[3 4]  OutputSizes=1
  Selector2 : Selector  InputPortWidth=6  IndexOptions=Index vector (dialog)  Indices=[5 6]  OutputSizes=1
  Sum : Sum  Inputs=++|
  X_Predict : Outport
  wires:
  Rotation_Data/1 -> Bus Selector2/1
  Bus Selector2/1 -> Multiply/1  "<M_OB>"
  Multiply/1 -> Selector/1  "acc_O"
  Bus Selector2/2 -> Multiply/2  "<acc_B_mDs2>"
  X_Prio/1 -> Selector1/1, Sum/1, Selector2/1
  Selector/1 -> Add/2
  Selector1/1 -> Mux/1
  Constant/1 -> Mux/3
  Mux/1 -> Reshape/1
  Reshape/1 -> Gain/1
  Sum/1 -> X_Predict/1
  Gain/1 -> Sum/2
  Add/1 -> Mux/2
  Selector2/1 -> Add/1

== system INS/Data_Fusion/Translation_Filter/CF/Verticle_Filter/Correct/Baro_Correct ==
  X_Predict : Inport
  Processed_Data : Inport  Port=2
  Baro_Correct : Subsystem
  Bus Selector : BusSelector  OutputSignals=Sensor_Enable.baro_enable
  Switch : Switch  Criteria=u2 > Threshold
  X_Next : Outport
  wires:
  Switch/1 -> X_Next/1
  Bus Selector/1 -> Baro_Correct/Enable, Switch/2  "<baro_enable>"
  Processed_Data/1 -> Baro_Correct/1(Processed_Data), Bus Selector/1
  Baro_Correct/1(X_Next) -> Switch/1
  X_Predict/1 -> Baro_Correct/2(X_Predict), Switch/3

== system INS/Data_Fusion/Translation_Filter/CF/Verticle_Filter/Correct/GPS_Correct ==
  X_Predict : Inport
  Processed_Data : Inport  Port=2
  Bus Selector : BusSelector  OutputSignals=Sensor_Enable.gps_height_enable
  GPS_Correct : Subsystem
  Switch : Switch  Criteria=u2 > Threshold
  X_Next : Outport
  wires:
  Switch/1 -> X_Next/1
  Bus Selector/1 -> GPS_Correct/Enable, Switch/2  "<gps_height_enable>"
  Processed_Data/1 -> GPS_Correct/1(Processed_Data), Bus Selector/1
  GPS_Correct/1(X_Next) -> Switch/1
  X_Predict/1 -> GPS_Correct/2(X_Predict), Switch/3

== system INS/Data_Fusion/Translation_Filter/CF/Verticle_Filter/Predict/Propagate ==
  X_Prio : Inport
  Processed_Data : Inport  Port=2
  Bus Selector : BusSelector  OutputSignals=Init_Condition.height_reset
  Delay : Delay  DelayLength=1
  States_Init : Subsystem
  Switch : Switch  Criteria=u2 > Threshold
  X : Outport
  wires:
  X_Prio/1 -> Delay/1
  Processed_Data/1 -> States_Init/1(Processed_Data), Bus Selector/1
  Bus Selector/1 -> Switch/2  "<height_reset>"
  Switch/1 -> X/1
  States_Init/1(X_0) -> Switch/1
  Delay/1 -> Switch/3

== system INS/Data_Fusion/Translation_Filter/CF/Verticle_Filter/Predict/Update ==
  X_Prio : Inport
  Rotation_Data : Inport  Port=2
  Add : Sum  Inputs=-++
  Bus Selector2 : BusSelector  OutputSignals=M_OB,acc_B_mDs2
  Constant : Constant  Value=0  OutDataTypeStr=single
  Constant1 : Constant  Value=INS_CONST.g  OutDataTypeStr=single
  Gain : Gain  Gain=INS_CONST.dt  OutDataTypeStr=Inherit: Same as input
  Gain1 : Gain  Gain=-1  OutDataTypeStr=Inherit: Same as input
  Multiply : Product  Multiplication=Matrix(*)
  Mux : Mux  Inputs=3
  Reshape : Reshape  OutputDimensionality=Customize  OutputDimensions=[3,1]
  Selector : Selector  InputPortWidth=3  IndexOptions=Index vector (dialog)  Indices=[3]  OutputSizes=1
  Selector1 : Selector  InputPortWidth=3  IndexOptions=Index vector (dialog)  Indices=[2]  OutputSizes=1
  Selector2 : Selector  InputPortWidth=3  IndexOptions=Index vector (dialog)  Indices=[3]  OutputSizes=1
  Sum : Sum  Inputs=++|
  X_Predict : Outport
  wires:
  Rotation_Data/1 -> Bus Selector2/1
  Bus Selector2/1 -> Multiply/1  "<M_OB>"
  Multiply/1 -> Selector/1  "acc_O"
  Bus Selector2/2 -> Multiply/2  "<acc_B_mDs2>"
  X_Prio/1 -> Selector2/1, Sum/1, Selector1/1
  Selector/1 -> Add/2
  Selector1/1 -> Gain1/1
  Constant/1 -> Mux/3
  Mux/1 -> Reshape/1
  Reshape/1 -> Gain/1
  Sum/1 -> X_Predict/1
  Add/1 -> Mux/2
  Constant1/1 -> Add/3
  Selector2/1 -> Add/1  "bias_az"
  Gain1/1 -> Mux/1
  Gain/1 -> Sum/2

== system INS/Data_Fusion/Translation_Filter/Process/Process_Data/Init_Condition/Bus_Selection ==
  Sensor_Meas : Inport
  Bus Selector1 : BusSelector  OutputSignals=GPS_Meas.dx_dmue,GPS_Meas.dy_dlambda,GPS_Meas.dz_dh,GPS_Meas.mue_rad,GPS_Meas.lambda_rad,GPS_Meas.h_m
  Mux : Mux  Inputs=3
  Mux1 : Mux  Inputs=3
  WGS84_derivatives : Outport
  WGS84_position : Outport  Port=2
  wires:
  Mux1/1 -> WGS84_position/1
  Sensor_Meas/1 -> Bus Selector1/1
  Mux/1 -> WGS84_derivatives/1
  Bus Selector1/6 -> Mux1/3  "<h_m>"
  Bus Selector1/5 -> Mux1/2  "<lambda_rad>"
  Bus Selector1/4 -> Mux1/1  "<mue_rad>"
  Bus Selector1/3 -> Mux/3  "<dz_dh>"
  Bus Selector1/2 -> Mux/2  "<dy_dlambda>"
  Bus Selector1/1 -> Mux/1  "<dx_dmue>"

== system INS/Data_Fusion/Translation_Filter/Process/Process_Data/Init_Condition/Pos_Reset ==
  Rotation_Data : Inport
  global_reset : Inport  Port=2
  Validity : Inport  Port=3
  Height_Reset : Subsystem
  Position_Reset : Subsystem
  pos_reset : Outport
  height_reset : Outport  Port=2
  wires:
  Rotation_Data/1 -> Height_Reset/1(Rotation_Data), Position_Reset/1(Rotation_Data)
  Validity/1 -> Height_Reset/2(Validity), Position_Reset/2(Validity)
  global_reset/1 -> Height_Reset/3(global_reset), Position_Reset/3(global_reset)
  Position_Reset/1(pos_reset) -> pos_reset/1
  Height_Reset/1(height_reset) -> height_reset/1

== system INS/Data_Fusion/Translation_Filter/Process/Process_Data/Init_Condition/WGS84_Reference ==
  Validity : Inport
  Translation_Data : Inport  Port=2
  WGS84_derivatives : Inport  Port=3
  WGS84_position : Inport  Port=4
  Bus_Assignment : Subsystem
  WGS84_Height_Ref : Subsystem
  WGS84_Position_Ref : Subsystem
  WGS84_Ref : Outport
  wires:
  WGS84_position/1 -> WGS84_Position_Ref/1(WGS84_position), WGS84_Height_Ref/1(WGS84_position)
  Translation_Data/1 -> WGS84_Position_Ref/2(Translation_Data), WGS84_Height_Ref/2(Translation_Data)
  Validity/1 -> WGS84_Position_Ref/3(Validity), WGS84_Height_Ref/3(Validity)
  WGS84_derivatives/1 -> WGS84_Position_Ref/4(WGS84_derivatives), WGS84_Height_Ref/4(WGS84_derivatives)
  WGS84_Position_Ref/1(WGS84_pos_ref) -> Bus_Assignment/1(WGS84_pos_ref)
  WGS84_Position_Ref/2(WGS84_dpos_ref) -> Bus_Assignment/2(WGS84_dpos_ref)
  WGS84_Height_Ref/1(WGS84_hgt_ref) -> Bus_Assignment/3(WGS84_hgt_ref)
  WGS84_Height_Ref/2(WGS84_dhgt_ref) -> Bus_Assignment/4(WGS84_dhgt_ref)
  Bus_Assignment/1(WGS84_Ref) -> WGS84_Ref/1

== system INS/Data_Fusion/Translation_Filter/Process/Process_Data/Sensor_Enable/Sensor_Horizontal_Select ==
  gps_pos_quality : Inport
  gps_spd_quality : Inport  Port=2
  gps_valid : Inport  Port=3
  opt_flow_valid : Inport  Port=4
  Compare To Zero : simulink/Logic and Bit Operations/Compare To Zero  relop=>  OutDataTypeStr=boolean
  Compare To Zero1 : simulink/Logic and Bit Operations/Compare To Zero  relop=>  OutDataTypeStr=boolean
  Compare To Zero2 : simulink/Logic and Bit Operations/Compare To Zero  relop=>  OutDataTypeStr=boolean
  Logical Operator : Logic  AllPortsSameDT=off  OutDataTypeStr=boolean
  Max : MinMax  Function=max  Inputs=2
  Min : MinMax
  Signal Copy : SignalConversion  OverrideOpt=off
  gps_enable : Outport
  op_flow_enable : Outport  Port=2
  wires:
  gps_pos_quality/1 -> Compare To Zero/1
  Compare To Zero/1 -> Max/2
  gps_valid/1 -> Logical Operator/1
  Logical Operator/1 -> Min/1
  opt_flow_valid/1 -> Signal Copy/1
  gps_spd_quality/1 -> Compare To Zero1/1
  Compare To Zero1/1 -> Max/1
  Max/1 -> Logical Operator/2
  Min/1 -> Compare To Zero2/1
  Compare To Zero2/1 -> gps_enable/1
  Signal Copy/1 -> op_flow_enable/1

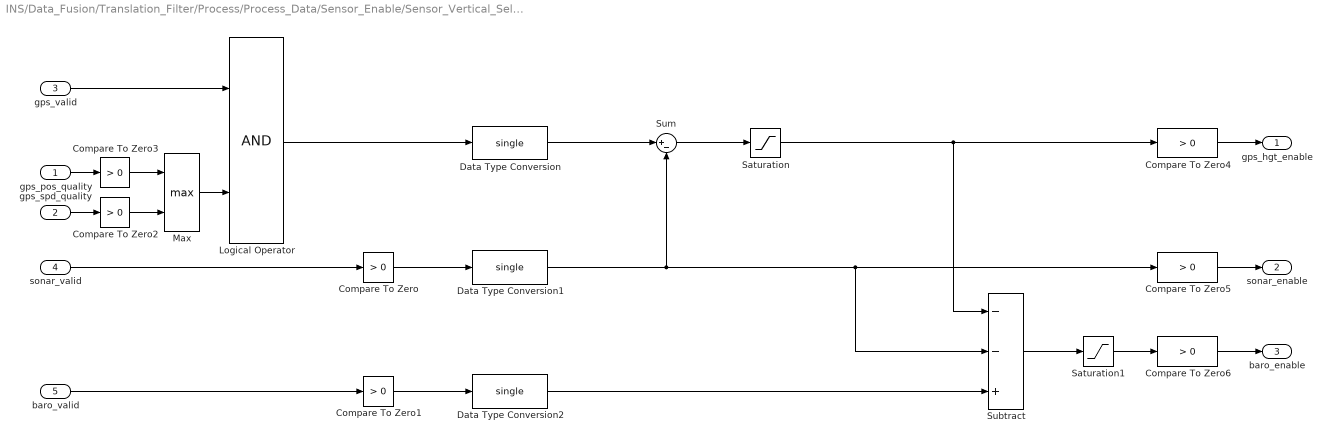
== system INS/Data_Fusion/Translation_Filter/Process/Process_Data/Sensor_Enable/Sensor_Vertical_Select ==
  gps_pos_quality : Inport
  gps_spd_quality : Inport  Port=2
  gps_valid : Inport  Port=3
  sonar_valid : Inport  Port=4
  baro_valid : Inport  Port=5
  Compare To Zero{,1..6} (7 alike) : simulink/Logic and Bit Operations/Compare To Zero  relop=>  OutDataTypeStr=boolean
  Data Type Conversion : DataTypeConversion  OutDataTypeStr=single
  Data Type Conversion1 : DataTypeConversion  OutDataTypeStr=single
  Data Type Conversion2 : DataTypeConversion  OutDataTypeStr=single
  Logical Operator : Logic  AllPortsSameDT=off  OutDataTypeStr=boolean
  Max : MinMax  Function=max  Inputs=2
  Saturation : Saturate  UpperLimit=1  LowerLimit=0
  Saturation1 : Saturate  UpperLimit=1  LowerLimit=0
  Subtract : Sum  Inputs=--+
  Sum : Sum  Inputs=|+-
  gps_hgt_enable : Outport
  sonar_enable : Outport  Port=2
  baro_enable : Outport  Port=3
  wires:
  Data Type Conversion1/1 -> Subtract/2, Compare To Zero5/1, Sum/2
  Compare To Zero/1 -> Data Type Conversion1/1
  sonar_valid/1 -> Compare To Zero/1
  Sum/1 -> Saturation/1
  Logical Operator/1 -> Data Type Conversion/1
  Saturation/1 -> Compare To Zero4/1, Subtract/1
  gps_pos_quality/1 -> Compare To Zero3/1
  Data Type Conversion/1 -> Sum/1
  baro_valid/1 -> Compare To Zero1/1
  Compare To Zero1/1 -> Data Type Conversion2/1
  Subtract/1 -> Saturation1/1
  Saturation1/1 -> Compare To Zero6/1
  Data Type Conversion2/1 -> Subtract/3
  Max/1 -> Logical Operator/2
  Compare To Zero2/1 -> Max/2
  Compare To Zero3/1 -> Max/1
  gps_valid/1 -> Logical Operator/1
  gps_spd_quality/1 -> Compare To Zero2/1
  Compare To Zero4/1 -> gps_hgt_enable/1
  Compare To Zero5/1 -> sonar_enable/1
  Compare To Zero6/1 -> baro_enable/1

== system INS/Data_Fusion/Translation_Filter/Process/Process_Data/Sensor_Valid/Position_Validity ==
  Sensor_Status : Inport
  Horizontal_Validity : Subsystem
  Vertical_Validity : Subsystem
  lon_lat_valid : Outport
  xy_R_valid : Outport  Port=2
  altitude_valid : Outport  Port=3
  h_R_valid : Outport  Port=4
  wires:
  Sensor_Status/1 -> Vertical_Validity/1(Sensor_Status), Horizontal_Validity/1(Sensor_Status)
  Horizontal_Validity/1(WGS84_pos_valid) -> lon_lat_valid/1
  Horizontal_Validity/2(xy_R_valid) -> xy_R_valid/1
  Vertical_Validity/2(h_R_valid) -> h_R_valid/1
  Vertical_Validity/1(WGS84_height_valid) -> altitude_valid/1

== system INS/Sensor_Process/Mag_Process/Magnetometer/Quality_Indication/Mag_Quality_Estimate/Inclination_Quality_Estimate ==
  nominal_inc_deg : Inport
  mag_normalized_O : Inport  Port=2
  Abs1 : Abs
  Constant2 : Constant  OutDataTypeStr=Inherit: Inherit via back propagation
  Gain1 : Gain  Gain=pi/180
  Saturation : Saturate  UpperLimit=1  LowerLimit=0
  Selector : Selector  InputPortWidth=3  IndexOptions=Index vector (dialog)  Indices=[1 2]  OutputSizes=1
  Selector1 : Selector  InputPortWidth=3  IndexOptions=Index vector (dialog)  Indices=3  OutputSizes=1
  Subtract : Sum  Inputs=+-
  Sum3 : Sum  Inputs=+-|
  Trigonometric Function : Trigonometry  Operator=atan2
  gain : Gain  Gain=2
  vec_modulus : AP_Math/vec_modulus  SystemSampleTime=-1
  inclination_quality : Outport
  wires:
  mag_normalized_O/1 -> Selector1/1, Selector/1
  Trigonometric Function/1 -> Subtract/2  "Inclination"
  vec_modulus/1 -> Trigonometric Function/2
  Abs1/1 -> gain/1  "inclination_error"
  gain/1 -> Sum3/2
  Gain1/1 -> Subtract/1  "nominal_inc"
  Subtract/1 -> Abs1/1
  Constant2/1 -> Sum3/1
  nominal_inc_deg/1 -> Gain1/1
  Sum3/1 -> Saturation/1
  Selector/1 -> vec_modulus/1
  Selector1/1 -> Trigonometric Function/1
  Saturation/1 -> inclination_quality/1

== system INS/Sensor_Process/Mag_Process/Magnetometer/Quality_Indication/Mag_Quality_Estimate/Intensity_Quality_Estimate ==
  mag_normalized_O : Inport
  Abs : Abs
  Constant1 : Constant  OutDataTypeStr=Inherit: Inherit via back propagation
  Nominal_Magnitude : Constant  OutDataTypeStr=Inherit: Inherit via back propagation
  Saturation : Saturate  UpperLimit=1  LowerLimit=0
  Subtract : Sum  Inputs=+-
  Sum : Sum  Inputs=+-|
  gain : Gain
  vec_modulus : AP_Math/vec_modulus  SystemSampleTime=-1
  intensity_quality : Outport
  wires:
  Constant1/1 -> Sum/1
  vec_modulus/1 -> Subtract/2
  Subtract/1 -> Abs/1
  Sum/1 -> Saturation/1
  mag_normalized_O/1 -> vec_modulus/1
  Nominal_Magnitude/1 -> Subtract/1
  Saturation/1 -> intensity_quality/1
  Abs/1 -> gain/1  "magnitude_error"
  gain/1 -> Sum/2

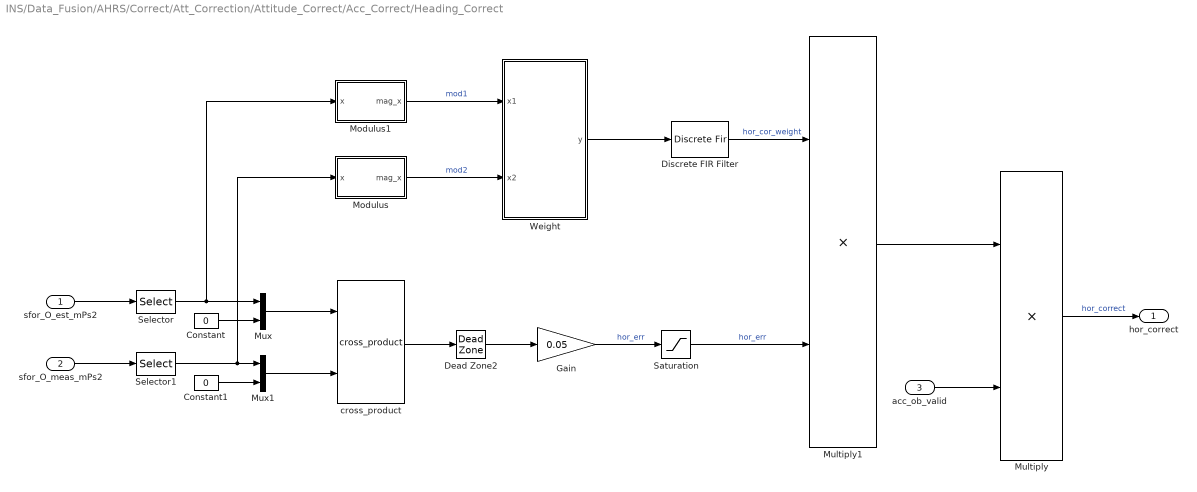
== system INS/Data_Fusion/AHRS/Correct/Att_Correction/Attitude_Correct/Acc_Correct/Heading_Correct ==
  sfor_O_est_mPs2 : Inport
  sfor_O_meas_mPs2 : Inport  Port=2
  acc_ob_valid : Inport  Port=3
  Constant : Constant  Value=0  OutDataTypeStr=single
  Constant1 : Constant  Value=0  OutDataTypeStr=single
  Dead Zone2 : DeadZone  LowerValue=-0.2  UpperValue=0.2  SaturateOnIntegerOverflow=on
  Discrete FIR Filter : DiscreteFir  Coefficients=ones(1,30)/30
  Gain : Gain  Gain=0.05  OutDataTypeStr=single
  Modulus : Subsystem
  Modulus1 : Subsystem
  Multiply : Product
  Multiply1 : Product
  Mux : Mux  Inputs=2
  Mux1 : Mux  Inputs=2
  Saturation : Saturate
  Selector : Selector  InputPortWidth=3  IndexOptions=Index vector (dialog)  Indices=[1 2]  OutputSizes=1
  Selector1 : Selector  InputPortWidth=3  IndexOptions=Index vector (dialog)  Indices=[1 2]  OutputSizes=1
  Weight : Subsystem
  cross_product : AP_Math/cross_product  SystemSampleTime=-1
  hor_correct : Outport
  wires:
  Dead Zone2/1 -> Gain/1
  Saturation/1 -> Multiply1/2  "hor_err"
  Mux1/1 -> cross_product/2
  Mux/1 -> cross_product/1
  sfor_O_meas_mPs2/1 -> Selector1/1
  Discrete FIR Filter/1 -> Multiply1/1  "hor_cor_weight"
  Weight/1(y) -> Discrete FIR Filter/1
  cross_product/1 -> Dead Zone2/1
  Modulus/1(mag_x) -> Weight/2(x2)  "mod2"
  Modulus1/1(mag_x) -> Weight/1(x1)  "mod1"
  Selector/1 -> Mux/1, Modulus1/1(x)
  Constant/1 -> Mux/2
  sfor_O_est_mPs2/1 -> Selector/1
  Multiply1/1 -> Multiply/1
  Selector1/1 -> Mux1/1, Modulus/1(x)
  Constant1/1 -> Mux1/2
  acc_ob_valid/1 -> Multiply/2
  Multiply/1 -> hor_correct/1  "hor_correct"
  Gain/1 -> Saturation/1  "hor_err"

== system INS/Data_Fusion/AHRS/Correct/Att_Correction/Attitude_Correct/Acc_Correct/Verticle_Correct ==
  acc_est_O_mPs2 : Inport
  acc_meas_O_mPs2 : Inport  Port=2
  Constant8 : Constant  Value=10/180*pi  OutDataTypeStr=single
  Cross_Product2 : Subsystem
      mask help: Cross Product
      mask Help: Cross Product
      mask Display: disp('y = u x v');
  Gain : Gain  Gain=[0.2;0.2;0]
  NonlinerSaturation : Subsystem
  vec_normalize : AP_Math/vec_normalize  SystemSampleTime=-1
  vec_normalize1 : AP_Math/vec_normalize  SystemSampleTime=-1
  vert_correct : Outport
  wires:
  NonlinerSaturation/1(y) -> Gain/1
  Cross_Product2/1(axb) -> NonlinerSaturation/1(u)
  vec_normalize/1 -> Cross_Product2/1(a)
  acc_meas_O_mPs2/1 -> vec_normalize1/1
  Gain/1 -> vert_correct/1
  acc_est_O_mPs2/1 -> vec_normalize/1
  vec_normalize1/1 -> Cross_Product2/2(b)
  Constant8/1 -> NonlinerSaturation/2(lim)

== system INS/Data_Fusion/AHRS/Correct/Att_Correction/Attitude_Correct/Measured_Acc/GPS_Acc_Observer ==
  reset : Inport
  GPS_vel_O_mPs : Inport  Port=2
  Enable : EnablePort  StatesWhenEnabling=reset
  ContinueLinearObserver : Subsystem  mask{wn=10, ksi=0.707}
      mask prompts: wn "Cut frequency (rad/s)"; ksi "Damping ratio"
  Terminator1 : Terminator
  GPS_acc_O_mPs2 : Outport
  wires:
  GPS_vel_O_mPs/1 -> ContinueLinearObserver/1(xr)
  ContinueLinearObserver/1(x1) -> Terminator1/1
  reset/1 -> ContinueLinearObserver/2(reset)
  ContinueLinearObserver/2(x2) -> GPS_acc_O_mPs2/1

== system INS/Data_Fusion/AHRS/Correct/Att_Correction/Attitude_Correct/Measured_Acc/Observer_Sensor ==
  Sensor_Data : Inport
  Bus Selector : BusSelector  OutputSignals=GPS_Data.GPS_reset,GPS_Data.sqd_quality
  Bus Selector1 : BusSelector  OutputSignals=VisionFlow_Data.valid
  Bus Selector2 : BusSelector  OutputSignals=GPS_Data.vn_mPs,GPS_Data.ve_mPs,GPS_Data.vd_mPs
  Bus Selector3 : BusSelector  OutputSignals=VisionFlow_Data.vel_x_O_mDs,VisionFlow_Data.vel_y_O_mDs
  Constant : Constant  Value=0  OutDataTypeStr=single
  Logical Operator : Logic  Operator=NOT  AllPortsSameDT=off  OutDataTypeStr=boolean
  Logical Operator1 : Logic  AllPortsSameDT=off  OutDataTypeStr=boolean
  Mux : Mux  Inputs=3
  Mux1 : Mux  Inputs=3
  Relay : Relay  OnSwitchValue=0.2  OffSwitchValue=0.1
  Saturation : Saturate  UpperLimit=1  LowerLimit=0
  Sum : Sum  Inputs=-+|
  gps_ob_enable : Outport
  GPS_vel_O_mPs : Outport  Port=2
  opt_flow_ob_enable : Outport  Port=3
  opt_flow_vel_O_mPs : Outport  Port=4
  wires:
  Mux/1 -> GPS_vel_O_mPs/1
  Bus Selector2/3 -> Mux/3  "<vd_mPs>"
  Bus Selector2/2 -> Mux/2  "<ve_mPs>"
  Bus Selector2/1 -> Mux/1  "<vn_mPs>"
  Logical Operator/1 -> Logical Operator1/1
  Sensor_Data/1 -> Bus Selector/1, Bus Selector3/1, Bus Selector2/1, Bus Selector1/1
  Logical Operator1/1 -> Sum/1, gps_ob_enable/1
  Bus Selector/1 -> Logical Operator/1  "<GPS_reset>"
  Relay/1 -> Logical Operator1/2
  Bus Selector/2 -> Relay/1  "<sqd_quality>"
  Bus Selector1/1 -> Sum/2  "<valid>"
  Bus Selector3/1 -> Mux1/1  "<vel_x_O_mDs>"
  Bus Selector3/2 -> Mux1/2  "<vel_y_O_mDs>"
  Constant/1 -> Mux1/3
  Mux1/1 -> opt_flow_vel_O_mPs/1
  Sum/1 -> Saturation/1
  Saturation/1 -> opt_flow_ob_enable/1

== system INS/Data_Fusion/AHRS/Correct/Att_Correction/Attitude_Correct/Measured_Acc/OpticalFlow_Acc_Observer ==
  OptFlow_vel_O_mDs : Inport
  Enable : EnablePort  StatesWhenEnabling=reset
  Constant : Constant  Value=0  OutDataTypeStr=single
  ContinueLinearObserver : Subsystem  mask{wn=10, ksi=0.707}
      mask prompts: wn "Cut frequency (rad/s)"; ksi "Damping ratio"
  Mux : Mux  Inputs=2
  Reshape : Reshape  OutputDimensionality=Customize  OutputDimensions=[3,1]
  Selector : Selector  InputPortWidth=3  IndexOptions=Index vector (dialog)  Indices=[1 2]  OutputSizes=1
  Terminator : Terminator
  OptFlow_acc_O_mPs2 : Outport
  wires:
  Mux/1 -> Reshape/1
  OptFlow_vel_O_mDs/1 -> Selector/1
  Constant/1 -> Mux/2
  ContinueLinearObserver/2(x2) -> Mux/1
  ContinueLinearObserver/1(x1) -> Terminator/1
  Selector/1 -> ContinueLinearObserver/1(xr)
  Reshape/1 -> OptFlow_acc_O_mPs2/1
